simulink model "Cruise_Control_Design"  (R2025b)
settings: Solver=VariableStepAuto  StartTime=0.0  StopTime=80  FixedStep=0.01  RelTol=1e-3
model workspace (MAT data in the model file):
  A = Simulink.Parameter
  A.Value = 2.2
  A.Complexity = 'real'
  A.Dimensions = [1 1]
  A.DataType = 'auto'
  Cd = Simulink.Parameter
  Cd.Value = 0.15
  Cd.Complexity = 'real'
  Cd.Dimensions = [1 1]
  Cd.DataType = 'auto'
  b = Simulink.Parameter
  b.Value = 10
  b.Complexity = 'real'
  b.Dimensions = [1 1]
  b.DataType = 'auto'
  g = Simulink.Parameter
  g.Value = 9.81
  g.Complexity = 'real'
  g.Dimensions = [1 1]
  g.DataType = 'auto'
  m = Simulink.Parameter
  m.Value = 1000
  m.Complexity = 'real'
  m.Dimensions = [1 1]
  m.DataType = 'auto'
  rho = Simulink.Parameter
  rho.Value = 1.225
  rho.Complexity = 'real'
  rho.Dimensions = [1 1]
  rho.DataType = 'auto'
libraries: SignalEditorBlockLib x1, slpidlib x1, simulink_extras x1
settings Model: PacingRate=1.100000  Creator=Snide  LastModifiedBy=Snide

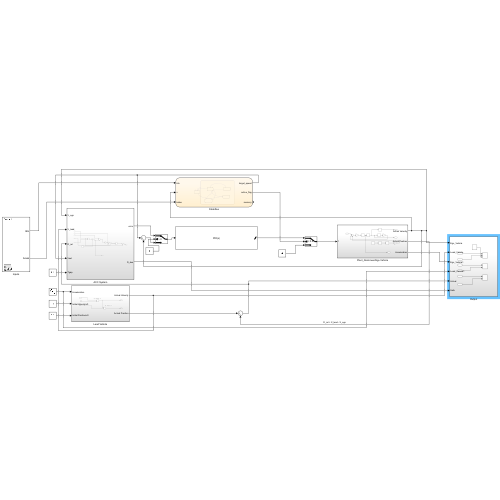
[thumbnail: Simulink's stored preview of the top-level diagram]
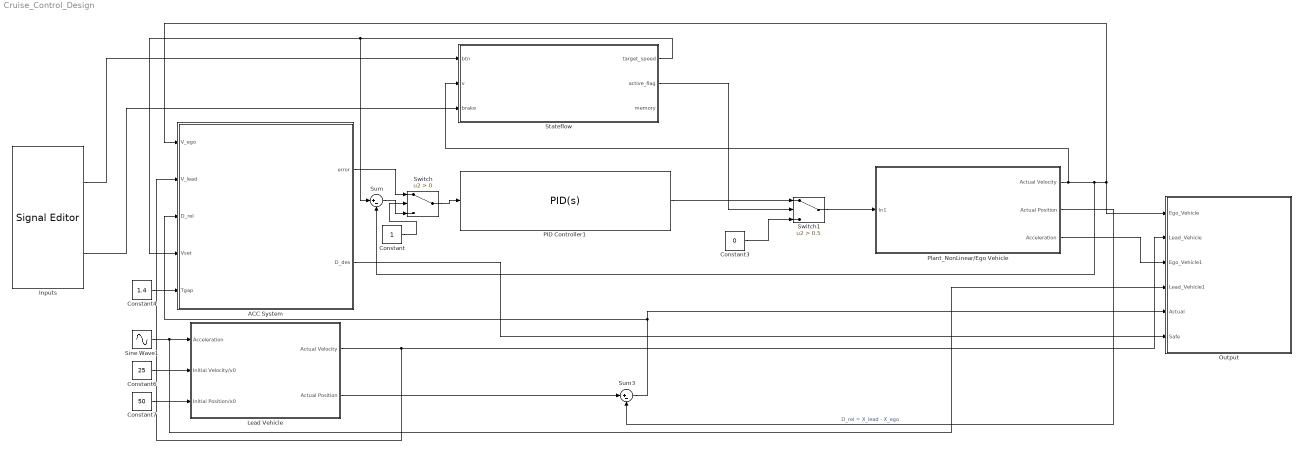
== system Cruise_Control_Design ==
  ACC System : Subsystem
  Constant : Constant
  Constant3 : Constant  Value=0  SampleTime=-1
  Constant4 : Constant  Value=1.4
  Constant6 : Constant  Value=25
  Constant7 : Constant  Value=50
  Inputs : SignalEditorBlockLib/Signal Editor  FileName=DataPoints.mat  ActiveScenario=Scenario  ActiveSignal=Btn  IsBus=off  OutputBusObjectStr=Bus: BusObject  SampleTime=0  ZeroCross=off  OutputAfterFinalValue=Setting to zero  Unit=inherit  PreserveSignalName=on  ApplySigPropsToAllScenarios=on  ApplySigPropsToAllSignals=off  SignalPropertySource=Dialog parameters
  Lead Vehicle : Subsystem
  Output : Subsystem
  PID Controller1 : slpidlib/PID Controller  Controller=PID  Form=Parallel  TimeDomain=Continuous-time  UseExternalTs=off  SampleTime=-1  IntegratorMethod=Forward Euler  FilterMethod=Forward Euler  ControllerParametersSource=internal  P=370  I=3  UseKiTs=off  D=-340  UseExternalDerivativeSource=off  N=6  UseFilter=on  TunerSelectOption=Transfer Function Based (PID Tuner App)  InitialConditionSource=internal  InitialConditionForIntegrator=0  InitialConditionForFilter=0  DifferentiatorICPrevScaledInput=0  ExternalReset=none  TrackingMode=off  Kt=1  LimitOutput=on  SatLimitsSource=internal  UpperSaturationLimit=6000  LowerSaturationLimit=-6000  LinearizeAsGain=on  AntiWindupMode=back-calculation  Kb=1  LimitIntegrator=off  UpperIntegratorSaturationLimit=inf  LowerIntegratorSaturationLimit=-inf  POutMin=[]  POutMax=[]  IOutMin=[]  IOutMax=[]  DOutMin=[]  DOutMax=[]  NOutMin=[]  NOutMax=[]  SumOutMin=[]  SumOutMax=[]  SaturationOutMin=[]  SaturationOutMax=[]  PParamMin=[]  PParamMax=[]  IParamMin=[]  IParamMax=[]  DParamMin=[]  DParamMax=[]  NParamMin=[]  NParamMax=[]  KbParamMin=[]  KbParamMax=[]  KtParamMin=[]  KtParamMax=[]  KbOutMin=[]  KbOutMax=[]  KtOutMin=[]  KtOutMax=[]  IntegratorOutMin=[]  IntegratorOutMax=[]  FilterOutMin=[]  FilterOutMax=[]  SumI1OutMin=[]  SumI1OutMax=[]  SumI2OutMin=[]  SumI2OutMax=[]  SumI3OutMin=[]  SumI3OutMax=[]  SumI4OutMin=[]  SumI4OutMax=[]  SumDOutMin=[]  SumDOutMax=[]  DifferentiatorOutMin=[]  DifferentiatorOutMax=[]  FilterDiffOutCoefMin=[]  FilterDiffOutCoefMax=[]  ReciprocalOutMin=[]  ReciprocalOutMax=[]  SumDenOutMin=[]  SumDenOutMax=[]  SumNumOutMin=[]  SumNumOutMax=[]  DivideOutMin=[]  DivideOutMax=[]  UdiffTsProdOutMin=[]  UdiffTsProdOutMax=[]  NTsProdOutMin=[]  NTsProdOutMax=[]  UintegralTsProdOutMin=[]  UintegralTsProdOutMax=[]  UngainTsProdOutMin=[]  UngainTsProdOutMax=[]  ClampingZeroOutDataTypeStr=Inherit: Inherit via back propagation  ClampingZeroOutMin=[]  ClampingZeroOutMax=[]  FilterDenConstantOutDataTypeStr=Inherit: Inherit via back propagation  FilterDenConstantOutMin=[]  FilterDenConstantOutMax=[]  PCopyOutDataTypeStr=Inherit: Inherit via back propagation  PCopyOutMin=[]  PCopyOutMax=[]  NCopyOutDataTypeStr=Inherit: Inherit via back propagation  NCopyOutMin=[]  NCopyOutMax=[]  IntegratorContinuousStateAttributes=''  IntegratorStateMustResolveToSignalObject=off  IntegratorRTWStateStorageClass=Auto  FilterContinuousStateAttributes=''  FilterStateMustResolveToSignalObject=off  FilterRTWStateStorageClass=Auto  ParallelPVariant=InternalParameters  IdealPVariant=Disabled  IVariant=InternalParameters  DVariant=InternalParameters  IntegratorVariant=Continuous  SatVariant=Enabled  AWVariant=BackCalculation  PCopyVariant=Disabled  TRVariant=Disabled  FdbkBlocksVariant=Forward  IdealPFdbkVariant=Disabled  SatFdbkVariant=Disabled  DerivativeFilterVariant=ContFilter  NVariant=InternalParameters  NCopyVariant=Disabled  FilterICVariant=InternalICsFilter  IntegratorICVariant=InternalICs  ExternalResetVariant=Disabled  TRSumVariant=Passthrough  SumFdbkVariant=Disabled  SumVariant=Sum_PID  TsampFilterVariant=InternalTs  TsampNgainVariant=Passthrough  TsampIntegralVariant=Disabled_SignalSpec  ExternalSaturationOutDataTypeStr=Inherit: Same as second input  DerivativeSourceVariant=ErrorSignal  PreIntVariant=InternalPreInt
  Plant_NonLinear/Ego Vehicle : Subsystem
  Sine Wave1 : Sin  Amplitude=0.45  Frequency=2*pi*0.027  SampleTime=0
  Stateflow : Stateflow chart  TreatAsAtomicUnit=on
  Sum : Sum  Inputs=|+-
  Sum3 : Sum  Inputs=|+-
  Switch : Switch  Criteria=u2 > Threshold  SaturateOnIntegerOverflow=off  InputSameDT=off
  Switch1 : Switch  Criteria=u2 > Threshold  Threshold=0.5  SaturateOnIntegerOverflow=off  InputSameDT=off
  wires:
  Constant3/1 -> Switch1/3
  Stateflow/2(active_flag) -> Switch1/2
  Switch1/1 -> Plant_NonLinear/Ego Vehicle/1(In1)
  Lead Vehicle/1(Actual Velocity) -> ACC System/2(V_lead), Output/2(Lead_Vehicle)
  Lead Vehicle/2(Actual Position) -> Sum3/1
  Plant_NonLinear/Ego Vehicle/1(Actual Velocity) -> Stateflow/2(v), Sum/2, ACC System/1(V_ego), Output/1(Ego_Vehicle)
  Plant_NonLinear/Ego Vehicle/2(Actual Position) -> Sum3/2  "D_rel = X_lead - X_ego"
  Sum3/1 -> ACC System/3(D_rel), Output/5(Actual)
  Stateflow/1(target_speed) -> Sum/1, ACC System/4(Vset)
  Constant4/1 -> ACC System/5(Tgap)
  Sine Wave1/1 -> Output/4(Lead_Vehicle1), Lead Vehicle/1(Acceleration)
  Constant6/1 -> Lead Vehicle/2(Initial Velocity/v0)
  Constant7/1 -> Lead Vehicle/3(Initial Position/x0)
  Inputs/1 -> Stateflow/1(btn)
  Inputs/2 -> Stateflow/3(brake)
  Plant_NonLinear/Ego Vehicle/3(Acceleration) -> Output/3(Ego_Vehicle1)
  ACC System/2(D_des) -> Output/6(Safe)
  PID Controller1/1 -> Switch1/1
  ACC System/1(error) -> Switch/1
  Sum/1 -> Switch/3
  Switch/1 -> PID Controller1/1
  Constant/1 -> Switch/2

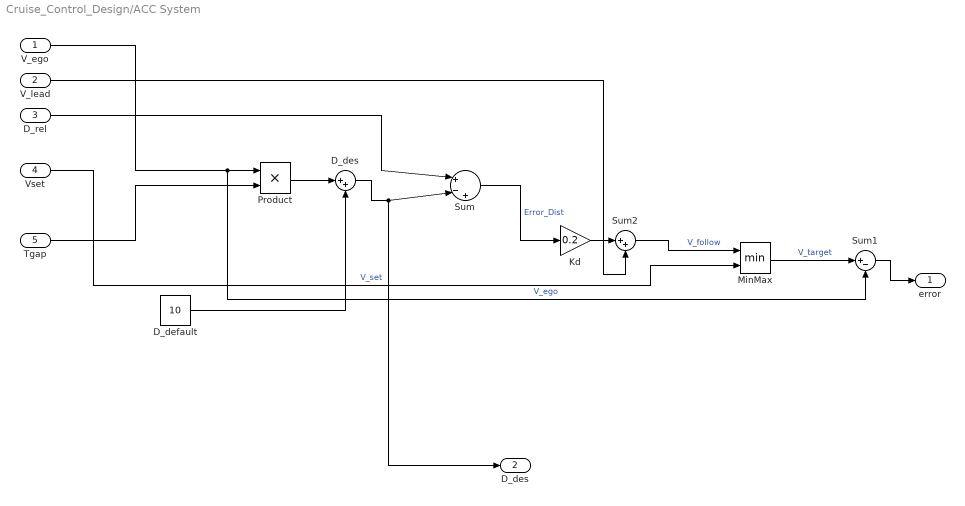
== system Cruise_Control_Design/ACC System ==
  V_ego : Inport
  V_lead : Inport  Port=2
  D_rel : Inport  Port=3
  Vset : Inport  Port=4
  Tgap : Inport  Port=5
  "              D_des" : Sum  Inputs=|++
  D_default : Constant  Value=10
  Kd : Gain  Gain=0.2
  MinMax : MinMax  Inputs=2
  Product : Product
  Sum : Sum  Inputs=|+-+
  Sum1 : Sum  Inputs=|+-
  Sum2 : Sum  Inputs=|++
  error : Outport
  D_des : Outport  Port=2
  wires:
  Tgap/1 -> Product/2
  V_ego/1 -> Sum1/2, Product/1  "V_ego"
  Product/1 -> "              D_des"/1
  D_default/1 -> "              D_des"/2
  D_rel/1 -> Sum/1
  "              D_des"/1 -> D_des/1, Sum/2
  Sum/1 -> Kd/1  "Error_Dist"
  Kd/1 -> Sum2/1
  V_lead/1 -> Sum2/2
  Sum2/1 -> MinMax/1  "V_follow"
  Vset/1 -> MinMax/2  "V_set"
  MinMax/1 -> Sum1/1  "V_target"
  Sum1/1 -> error/1

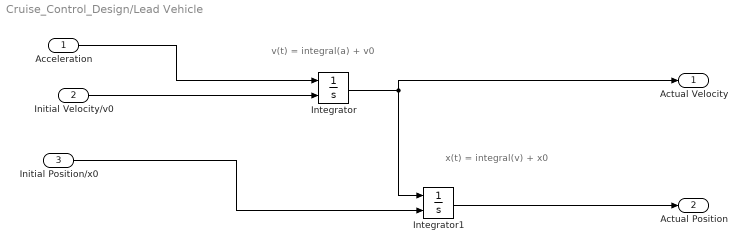
== system Cruise_Control_Design/Lead Vehicle ==
  note: v(t) = integral(a) + v0
  note: x(t) = integral(v) + x0
  Acceleration : Inport
  Initial Velocity/v0 : Inport  Port=2
  Initial Position/x0 : Inport  Port=3
  Integrator : Integrator  InitialConditionSource=external
  Integrator1 : Integrator  InitialConditionSource=external
  Actual Velocity : Outport
  Actual Position : Outport  Port=2  Unit=m
  wires:
  Acceleration/1 -> Integrator/1
  Integrator/1 -> Actual Velocity/1, Integrator1/1
  Integrator1/1 -> Actual Position/1
  Initial Velocity/v0/1 -> Integrator/2
  Initial Position/x0/1 -> Integrator1/2

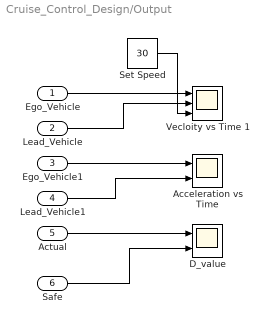
== system Cruise_Control_Design/Output ==
  Ego_Vehicle : Inport
  Lead_Vehicle : Inport  Port=2
  Ego_Vehicle1 : Inport  Port=3
  Lead_Vehicle1 : Inport  Port=4
  Actual : Inport  Port=5
  Safe : Inport  Port=6
  "Acceleration vs Time " : Scope  NumInputPorts=2
      settings: ActiveDisplayYMinimum=-3.6227831445199938  ActiveDisplayYMaximum=2.6050483006799436  DataLoggingVariableName=ScopeData6
  D_value : Scope  NumInputPorts=2
      settings: ActiveDisplayYMinimum=33.317217570106237  ActiveDisplayYMaximum=68.271607799326915  DataLoggingVariableName=ScopeData7
  Set Speed : Constant  Value=30
  Vecloity vs Time 1 : Scope  NumInputPorts=3
      settings: ActiveDisplayYMinimum=17.718450127771249  ActiveDisplayYMaximum=32.052924514546675  DataLoggingVariableName=ScopeData5
  wires:
  Ego_Vehicle/1 -> Vecloity vs Time 1/1
  Ego_Vehicle1/1 -> "Acceleration vs Time "/1
  Lead_Vehicle1/1 -> "Acceleration vs Time "/2
  Actual/1 -> D_value/1
  Safe/1 -> D_value/2
  Lead_Vehicle/1 -> Vecloity vs Time 1/2
  Set Speed/1 -> Vecloity vs Time 1/3

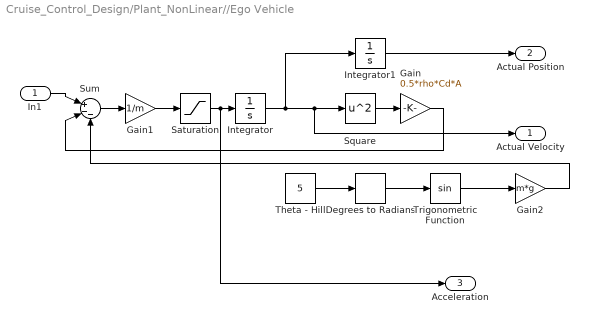
== system Cruise_Control_Design/Plant_NonLinear//Ego Vehicle ==
  In1 : Inport
  Degrees to Radians : simulink_extras/Transformations/Degrees to Radians
  Gain : Gain  Gain=0.5*rho*Cd*A
  Gain1 : Gain  Gain=1/m
  Gain2 : Gain  Gain=m*g
  Integrator : Integrator  InitialCondition=20  LowerSaturationLimit=0
  Integrator1 : Integrator  InitialCondition=10
  Saturation : Saturate  UpperLimit=2  LowerLimit=-3
  Square : Math  Operator=square
  Sum : Sum  Inputs=|+--
  Theta - Hill : Constant  Value=5
  Trigonometric Function : Trigonometry
  Actual Velocity : Outport
  Actual Position : Outport  Port=2  Unit=m
  Acceleration : Outport  Port=3
  wires:
  Square/1 -> Gain/1
  Gain/1 -> Sum/2
  Sum/1 -> Gain1/1
  In1/1 -> Sum/1
  Trigonometric Function/1 -> Gain2/1
  Gain2/1 -> Sum/3
  Integrator/1 -> Integrator1/1, Actual Velocity/1, Square/1
  Integrator1/1 -> Actual Position/1
  Gain1/1 -> Saturation/1
  Saturation/1 -> Acceleration/1, Integrator/1
  Degrees to Radians/1 -> Trigonometric Function/1
  Theta - Hill/1 -> Degrees to Radians/1

== stateflow chart Cruise_Control_Design/Stateflow ==
  state ON_MODE
    state SET
      en:
      stored_speed = 50;
      target_speed = 50;
      memory = v;
      active_flag = 1;
    state Accel
      du:
      target_speed = target_speed + 0.05;
      active_flag = 1;
    state Resume
      en:
      target_speed = stored_speed;
      active_flag = 1;
    state Deccel
      du:
      target_speed = target_speed - 0.05;
      active_flag = 1;
    Accel -> SET : [btn == 0]
    SET -> Accel [order 2] : [btn == 2]
    Deccel -> SET : [btn == 0]
    SET -> Deccel [order 1] : [btn == 3]
    Resume -> SET : [btn == 0]
  state OFF
    en:
    target_speed = 0;
    active_flag = 0;
  ON_MODE -> OFF : [brake == 1]
  OFF -> SET [order 2] : [btn == 1 && brake == 0]
  (default) -> OFF
  OFF -> Resume [order 1] : [btn == 4]
  data: btn input; v input; target_speed output; active_flag output; stored_speed local double =0; memory output; brake input
